simulink model "ControlLaws"  (R2020a)
settings: Solver=VariableStepAuto  StartTime=0.0  StopTime=10.0  RelTol=1e-3
values from neighbouring files (symbols this model uses):
  bp = 20    [ControlLawsScript.m]    (also in ControlLaws_Script.m = 0.001)
  bq = 0.001    [ControlLawsScript.m]    (also in ControlLaws_Script.m)
  br = 0.001    [ControlLawsScript.m]    (also in ControlLaws_Script.m)
  cx = 0.6    [ControlLawsScript.m]    (also in ControlLaws_Script.m = 5)
  cy = 0.005    [ControlLawsScript.m]    (also in ControlLaws_Script.m = 5)
  cz = 0.1    [ControlLawsScript.m]    (also in ControlLaws_Script.m = 5)
  g = 9.81    [ControlLawsScript.m]    (also in ControlLaws_Script.m = 9.80665; Qball_X8_Model.m = 9.87)
  Jx = 0.082298105960482    (= 0.0822981059605)    [ControlLawsScript.m]    (also in ControlLaws_Script.m)
  Jy = 0.082457201628499    (= 0.0824572016285)    [ControlLawsScript.m]    (also in ControlLaws_Script.m)
  Jz = 0.15887270137511    (= 0.158872701375)    [ControlLawsScript.m]    (also in ControlLaws_Script.m)
  Kp = (Jx/Tc)-bp    (= -17.942547351)    [ControlLawsScript.m]    (also in ControlLaws_Script.m = 4.11390529802)
  Kp2 = Jx*((4/ts))*((-4/ts)+((bp+Kp)/Jx))/Kp    (= -0.385287594088)    [ControlLawsScript.m]    (also in ControlLaws_Script.m = 6.72163348437)
  Kq = (Jy/Tc)-bq    (= 2.06043004071)    [ControlLawsScript.m]    (also in ControlLaws_Script.m = 4.12186008142)
  Kq2 = Jy*((4/ts))*((-4/ts)+((bq+Kq)/Jy))/Kq    (= 3.36163072753)    [ControlLawsScript.m]    (also in ControlLaws_Script.m = 6.72163033191)
  Kr = (Jz/Tc)-br    (= 3.97081753438)    [ControlLawsScript.m]    (also in ControlLaws_Script.m = 7.94263506876)
  Kr2 = Jz*((4/ts))*((-4/ts)+((br+Kr)/Jz))/Kr    (= 3.36084617336)    [ControlLawsScript.m]    (also in ControlLaws_Script.m = 6.72084606682)
  Kx1 = ((1/Tcxy)-cx)/g    (= 1.2130479103)    [ControlLawsScript.m]
  Kx2 = abs(Kx2)    [ControlLawsScript.m]
  Ky1 = ((1/Tcxy)-cy)/g    (= 1.27370030581)    [ControlLawsScript.m]
  Ky2 = abs(Ky2)    [ControlLawsScript.m]
  Kz = (m/Tcz)-cz    (= 43.4143536865)    [ControlLawsScript.m]    (also in ControlLaws_Script.m = 38.5143536865)
  Kz2 = m*((4/tsz))*((-4/tsz)+((cz+Kz)/m))/Kz    (= 1.68386968792)    [ControlLawsScript.m]    (also in ControlLaws_Script.m = 1.89810050529)
  m = 3.4811482949175    (= 3.48114829492)    [ControlLawsScript.m]    (also in ControlLaws_Script.m; Qball_X8_Model.m = 1.45)
  z_x = 4*(1+(1/(tan(t1+t2+t3-pi/4))))/ts2    [ControlLawsScript.m]    (also in ControlLaws_Script.m = 5)
  z_y = 4*(1+(1/(tan(ty_1+ty_2+ty_3-pi/4))))/ts2    [ControlLawsScript.m]    (also in ControlLaws_Script.m = 5)
settings Model: Creator=Asus  LastModifiedBy=alger
settings DebuggingCC: UnconnectedInputMsg=none  UnconnectedOutputMsg=none  UnconnectedLineMsg=none
settings ModelReferenceCC: EnableRefExpFcnMdlSchedulingChecks=off
settings RTWCC: Description=Generic Real-Time Target

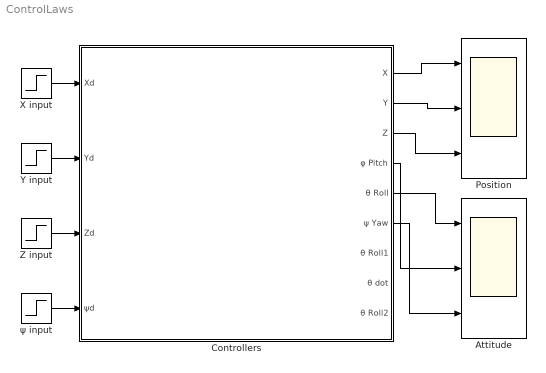
== system ControlLaws ==
  " Attitude" : Scope  NumInputPorts=3
  Controllers : Subsystem
  "Position " : Scope  NumInputPorts=3
  X input : Step  SampleTime=0
  Y input : Step  After=2  SampleTime=0
  Z input : Step  SampleTime=0
  ψ input : Step  Time=5  After=0.15  SampleTime=0
  wires:
  Controllers/2(Y) -> "Position "/2
  Controllers/3(Z) -> "Position "/3
  Controllers/6(ψ Yaw) -> " Attitude"/3
  ψ input/1 -> Controllers/4(ψd)
  Controllers/1(X) -> "Position "/1
  Y input/1 -> Controllers/2(Yd)
  Z input/1 -> Controllers/3(Zd)
  X input/1 -> Controllers/1(Xd)
  Controllers/4(φ Pitch) -> " Attitude"/2
  Controllers/5(θ Roll) -> " Attitude"/1

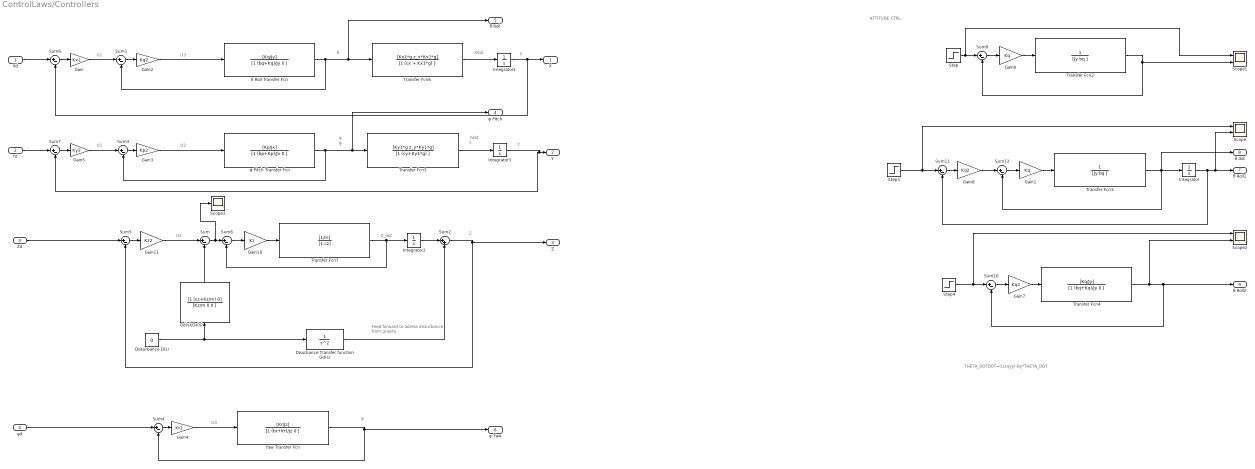
== system ControlLaws/Controllers ==
  note: THETA_DOTDOT=(U3/Jyy)-By*THETA_DOT
  note: ATTITUDE CTRL
  note: Feed forward to adress disturbance
      | from gravity
  note: φ
  note: U3
  note: U2
  note: U1
  note: U3
  note: Z_dot
  note: ψ
  note: Z
  note: Y
  note: ψ
  note: θ
  note: U1
  note: U1
  note: X
  note: Xdot
  note: Ydot
  note: Y
  Xd : Inport
  Yd : Inport  Port=2
  Zd : Inport  Port=3
  ψd : Inport  Port=4
  Disturbance D(s) : Constant  Value=g
  Disurbance Transfer function Gd(s) : TransferFcn  Denominator=[1 0 0 ]
  Gain : Gain  Gain=Kx2
  Gain1 : Gain  Gain=Kq
  Gain10 : Gain  Gain=Kz
  Gain11 : Gain  Gain=Kz2
  Gain2 : Gain  Gain=Kq2
  Gain3 : Gain  Gain=Kp2
  Gain4 : Gain  Gain=Kr2
  Gain5 : Gain  Gain=Ky2
  Gain6 : Gain  Gain=Kq
  Gain7 : Gain  Gain=Kq2
  Gain8 : Gain  Gain=Kq2
  Gd(s)/Gz(s) : TransferFcn  Numerator=[1 (cz+Kz/m) 0]  Denominator=[Kz/m 0 0 ]
  Integrator{,1..3} (4 alike) : Integrator
  Scope : Scope  NumInputPorts=2
  Scope1 : Scope  NumInputPorts=2
  Scope2 : Scope  NumInputPorts=2
  Scope3 : Scope
  Step : Step  SampleTime=0
  Step3 : Step  SampleTime=0
  Step4 : Step  After=5  SampleTime=0
  Sum{,1,3..12} (12 alike) : Sum  Inputs=|+-
  Sum2 : Sum  Inputs=|++
  Transfer Fcn1 : TransferFcn  Denominator=[Jy bq ]
  Transfer Fcn2 : TransferFcn  Denominator=[Jy bq ]
  Transfer Fcn3 : TransferFcn  Numerator=[Ky1*g z_y*Ky1*g]  Denominator=[1 (cy+Ky1*g) ]
  Transfer Fcn4 : TransferFcn  Numerator=[Kq/Jy]  Denominator=[1 (bq+Kq)/Jy 0 ]
  Transfer Fcn6 : TransferFcn  Numerator=[Kx1*g z_x*Kx1*g]  Denominator=[1 (cx + Kx1*g) ]
  Transfer Fcn7 : TransferFcn  Numerator=[1/m]  Denominator=[1 cz]
  "Yaw Transfer Fcn " : TransferFcn  Numerator=[Kr/Jz]  Denominator=[1 (br+Kr)/Jz 0 ]
  θ Roll Transfer Fcn : TransferFcn  Numerator=[Kq/Jy]  Denominator=[1 (bq+Kq)/Jy 0 ]
  φ Pitch Transfer Fcn : TransferFcn  Numerator=[Kp/Jx]  Denominator=[1 (bp+Kp)/Jx 0 ]
  X : Outport
  Y : Outport  Port=2
  Z : Outport  Port=3
  φ Pitch : Outport  Port=4
  θ Roll : Outport  Port=5
  ψ Yaw : Outport  Port=6
  θ Roll1 : Outport  Port=7
  θ dot : Outport  Port=8
  θ Roll2 : Outport  Port=9
  wires:
  Integrator3/1 -> Sum7/2, Y/1
  Sum7/1 -> Gain5/1
  Sum6/1 -> Gain/1
  Integrator1/1 -> Sum6/2, X/1
  Xd/1 -> Sum6/1
  Yd/1 -> Sum7/1
  θ Roll Transfer Fcn/1 -> Transfer Fcn6/1, θ Roll/1, Sum1/2
  φ Pitch Transfer Fcn/1 -> Transfer Fcn3/1, φ Pitch/1, Sum3/2
  "Yaw Transfer Fcn "/1 -> Sum4/2, ψ Yaw/1
  Gain/1 -> Sum1/1
  Sum1/1 -> Gain2/1
  Gain2/1 -> θ Roll Transfer Fcn/1
  Gain3/1 -> φ Pitch Transfer Fcn/1
  Gain4/1 -> "Yaw Transfer Fcn "/1
  Gain5/1 -> Sum3/1
  Sum3/1 -> Gain3/1
  Sum4/1 -> Gain4/1
  ψd/1 -> Sum4/1
  Gain10/1 -> Transfer Fcn7/1
  Sum8/1 -> Gain10/1
  Transfer Fcn7/1 -> Sum8/2, Integrator2/1
  Integrator2/1 -> Sum2/1
  Sum5/1 -> Gain11/1
  Zd/1 -> Sum5/1
  Gain11/1 -> Sum/1
  Sum/1 -> Scope3/1, Sum8/1
  Disturbance D(s)/1 -> Gd(s)/Gz(s)/1, Disurbance Transfer function Gd(s)/1
  Sum2/1 -> Sum5/2, Z/1
  Disurbance Transfer function Gd(s)/1 -> Sum2/2
  Gd(s)/Gz(s)/1 -> Sum/2
  Transfer Fcn6/1 -> Integrator1/1
  Transfer Fcn3/1 -> Integrator3/1
  Sum9/1 -> Gain6/1
  Transfer Fcn2/1 -> Scope1/2, Sum9/2
  Step/1 -> Sum9/1, Scope1/1
  Gain6/1 -> Transfer Fcn2/1
  Gain1/1 -> Transfer Fcn1/1
  Gain7/1 -> Transfer Fcn4/1
  Gain8/1 -> Sum12/1
  Sum11/1 -> Gain8/1
  Integrator/1 -> θ Roll1/1, Scope/2, Sum11/2
  Step3/1 -> Sum11/1, Scope/1
  Transfer Fcn4/1 -> Sum10/2, θ Roll2/1, Scope2/2
  Sum10/1 -> Gain7/1
  Step4/1 -> Scope2/1, Sum10/1
  Transfer Fcn1/1 -> Integrator/1, θ dot/1, Sum12/2
  Sum12/1 -> Gain1/1
